simulink model "wt_multi"  (R2022b)
settings: Solver=FixedStepDiscrete  StartTime=0.0  StopTime=10.0  RelTol=1e-3
PreLoadFcn:
  | addpath('/nfs/ug/homes-1/z/zha13325/ece1718/a2_k/a2_hw/hdlimport/wt_multi');
libraries: simulink x2808, hdlsllib x1459
(part 1 of 22)
CloseFcn:
  | addpath('/nfs/ug/homes-1/z/zha13325/ece1718/a2_k/a2_hw/hdlimport/wt_multi');
  | rmpath('/nfs/ug/homes-1/z/zha13325/ece1718/a2_k/a2_hw/hdlimport/wt_multi');
settings Model: DataTypeOverride=Off  Creator=zha13325  LastModifiedBy=zhangjx
settings OptimizationCC: BlockReduction=off  ConditionallyExecuteInputs=off  DefaultParameterBehavior=Inlined
settings DebuggingCC: AlgebraicLoopMsg=error  InheritedTsInSrcMsg=none  SingleTaskRateTransMsg=error  UnconnectedInputMsg=warning  UnconnectedOutputMsg=warning  UnconnectedLineMsg=warning
settings HardwareCC: ProdBitPerPointer=32  ProdBitPerSizeT=32  ProdBitPerPtrDiffT=32  ProdLargestAtomicFloat=None  ProdIntDivRoundTo=Undefined  ProdEndianess=Unspecified  ProdWordSize=32  ProdHWDeviceType=ASIC/FPGA->ASIC/FPGA  TargetBitPerLong=64  TargetBitPerPointer=64  TargetBitPerSizeT=64  TargetBitPerPtrDiffT=64  TargetLongLongMode=on  TargetIntDivRoundTo=Zero  TargetEndianess=LittleEndian  TargetWordSize=64  TargetHWDeviceType=Custom Processor->MATLAB Host Computer  ProdEqTarget=off
settings ModelReferenceCC: EnableRefExpFcnMdlSchedulingChecks=on
settings RTWCC: DLArmComputeVersion=19.05

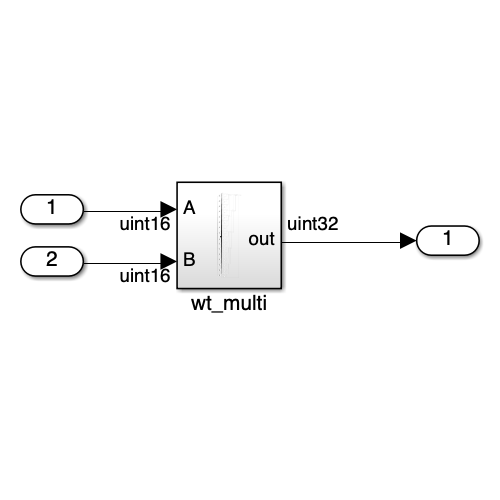
[thumbnail: Simulink's stored preview of the top-level diagram]
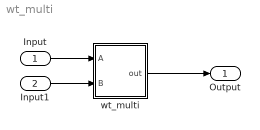
== system wt_multi ==
  Input : Inport
  Input1 : Inport  Port=2
  wt_multi : Subsystem
  Output : Outport
  wires:
  Input/1 -> wt_multi/1(A)
  Input1/1 -> wt_multi/2(B)
  wt_multi/1(out) -> Output/1

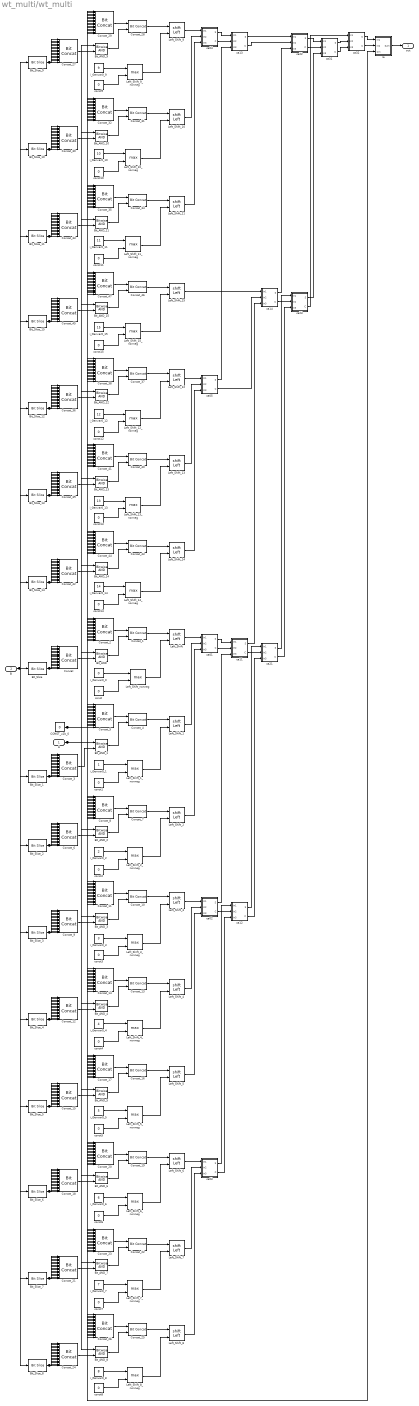
== system wt_multi/wt_multi ==
  A : Inport  OutDataTypeStr=uint16  SampleTime=-1
  B : Inport  Port=2  OutDataTypeStr=uint16  SampleTime=-1
  Bit_AND : simulink/Logic and Bit Operations/Bitwise Operator  logicop=AND  UseBitMask=off  NumInputPorts=2  BitMask=double(0)  BitMaskRealWorld=Real World Value
  Bit_AND_{1..15} (15 alike) : simulink/Logic and Bit Operations/Bitwise Operator  logicop=AND  UseBitMask=off  NumInputPorts=2  BitMask=double(0)  BitMaskRealWorld=Real World Value
  Bit_Slice : hdlsllib/Logic and Bit Operations/Bit Slice  lidx=double(0)  ridx=double(0)
  Bit_Slice_1 : hdlsllib/Logic and Bit Operations/Bit Slice  lidx=double(1)  ridx=double(1)
  Bit_Slice_10 : hdlsllib/Logic and Bit Operations/Bit Slice  lidx=double(10)  ridx=double(10)
  Bit_Slice_11 : hdlsllib/Logic and Bit Operations/Bit Slice  lidx=double(11)  ridx=double(11)
  Bit_Slice_12 : hdlsllib/Logic and Bit Operations/Bit Slice  lidx=double(12)  ridx=double(12)
  Bit_Slice_13 : hdlsllib/Logic and Bit Operations/Bit Slice  lidx=double(13)  ridx=double(13)
  Bit_Slice_14 : hdlsllib/Logic and Bit Operations/Bit Slice  lidx=double(14)  ridx=double(14)
  Bit_Slice_15 : hdlsllib/Logic and Bit Operations/Bit Slice  lidx=double(15)  ridx=double(15)
  Bit_Slice_2 : hdlsllib/Logic and Bit Operations/Bit Slice  lidx=double(2)  ridx=double(2)
  Bit_Slice_3 : hdlsllib/Logic and Bit Operations/Bit Slice  lidx=double(3)  ridx=double(3)
  Bit_Slice_4 : hdlsllib/Logic and Bit Operations/Bit Slice  lidx=double(4)  ridx=double(4)
  Bit_Slice_5 : hdlsllib/Logic and Bit Operations/Bit Slice  lidx=double(5)  ridx=double(5)
  Bit_Slice_6 : hdlsllib/Logic and Bit Operations/Bit Slice  lidx=double(6)  ridx=double(6)
  Bit_Slice_7 : hdlsllib/Logic and Bit Operations/Bit Slice  lidx=double(7)  ridx=double(7)
  Bit_Slice_8 : hdlsllib/Logic and Bit Operations/Bit Slice  lidx=double(8)  ridx=double(8)
  Bit_Slice_9 : hdlsllib/Logic and Bit Operations/Bit Slice  lidx=double(9)  ridx=double(9)
  CONST_u1b_0 : Constant  Value=0  OutDataTypeStr=fixdt(0, 1, 0)  SampleTime=-1
  Concat : hdlsllib/Logic and Bit Operations/Bit Concat  numInputs=16
  Concat_{1,4,7,10,13,16,19,22,25,28,31,34,37,40,43,46} (16 alike) : hdlsllib/Logic and Bit Operations/Bit Concat  numInputs=2
  Concat_{2..3,5..6,8..9,11..12,14..15,17..18,20..21,23..24,26..27,29..30,32..33,35..36,38..39,41..42,44..45,47} (31 alike) : hdlsllib/Logic and Bit Operations/Bit Concat  numInputs=16
  Left_Shift : ArithShift  BitShiftNumberSource=Input port  BitShiftDirection=Left
      settings: InputPortMap=u0,p1
  Left_Shift_{1..15} (15 alike) : ArithShift  BitShiftNumberSource=Input port  BitShiftDirection=Left
      settings: InputPortMap=u0,p1
  Left_Shift_10_nonneg : MinMax  Function=max  Inputs=2
  Left_Shift_11_nonneg : MinMax  Function=max  Inputs=2
  Left_Shift_12_nonneg : MinMax  Function=max  Inputs=2
  Left_Shift_13_nonneg : MinMax  Function=max  Inputs=2
  Left_Shift_14_nonneg : MinMax  Function=max  Inputs=2
  Left_Shift_15_nonneg : MinMax  Function=max  Inputs=2
  Left_Shift_1_nonneg : MinMax  Function=max  Inputs=2
  Left_Shift_2_nonneg : MinMax  Function=max  Inputs=2
  Left_Shift_3_nonneg : MinMax  Function=max  Inputs=2
  Left_Shift_4_nonneg : MinMax  Function=max  Inputs=2
  Left_Shift_5_nonneg : MinMax  Function=max  Inputs=2
  Left_Shift_6_nonneg : MinMax  Function=max  Inputs=2
  Left_Shift_7_nonneg : MinMax  Function=max  Inputs=2
  Left_Shift_8_nonneg : MinMax  Function=max  Inputs=2
  Left_Shift_9_nonneg : MinMax  Function=max  Inputs=2
  Left_Shift_nonneg : MinMax  Function=max  Inputs=2
  ca01 : Subsystem
  ca02 : Subsystem
  ca03 : Subsystem
  ca04 : Subsystem
  ca05 : Subsystem
  ca11 : Subsystem
  ca12 : Subsystem
  ca13 : Subsystem
  ca14 : Subsystem
  ca21 : Subsystem
  ca22 : Subsystem
  ca23 : Subsystem
  ca31 : Subsystem
  ca32 : Subsystem
  const{,1..15} (16 alike) : Constant  Value=0  OutDataTypeStr=int32  SampleTime=-1
  i_Genvar0_0 : Constant  Value=0  OutDataTypeStr=int32  SampleTime=-1
  i_Genvar0_1 : Constant  OutDataTypeStr=int32  SampleTime=-1
  i_Genvar0_10 : Constant  Value=10  OutDataTypeStr=int32  SampleTime=-1
  i_Genvar0_11 : Constant  Value=11  OutDataTypeStr=int32  SampleTime=-1
  i_Genvar0_12 : Constant  Value=12  OutDataTypeStr=int32  SampleTime=-1
  i_Genvar0_13 : Constant  Value=13  OutDataTypeStr=int32  SampleTime=-1
  i_Genvar0_14 : Constant  Value=14  OutDataTypeStr=int32  SampleTime=-1
  i_Genvar0_15 : Constant  Value=15  OutDataTypeStr=int32  SampleTime=-1
  i_Genvar0_2 : Constant  Value=2  OutDataTypeStr=int32  SampleTime=-1
  i_Genvar0_3 : Constant  Value=3  OutDataTypeStr=int32  SampleTime=-1
  i_Genvar0_4 : Constant  Value=4  OutDataTypeStr=int32  SampleTime=-1
  i_Genvar0_5 : Constant  Value=5  OutDataTypeStr=int32  SampleTime=-1
  i_Genvar0_6 : Constant  Value=6  OutDataTypeStr=int32  SampleTime=-1
  i_Genvar0_7 : Constant  Value=7  OutDataTypeStr=int32  SampleTime=-1
  i_Genvar0_8 : Constant  Value=8  OutDataTypeStr=int32  SampleTime=-1
  i_Genvar0_9 : Constant  Value=9  OutDataTypeStr=int32  SampleTime=-1
  ra : Subsystem
  out : Outport  OutDataTypeStr=uint32  SampleTime=-1
  wires:
  B/1 -> Bit_Slice_15/1, Bit_Slice_14/1, Bit_Slice_13/1, Bit_Slice_12/1, Bit_Slice_11/1, Bit_Slice_10/1, Bit_Slice_9/1, Bit_Slice_8/1, Bit_Slice_7/1, Bit_Slice_6/1, Bit_Slice_5/1, Bit_Slice_4/1, Bit_Slice_3/1, Bit_Slice_2/1, Bit_Slice_1/1, Bit_Slice/1
  Bit_Slice/1 -> Concat/16, Concat/15, Concat/14, Concat/13, Concat/12, Concat/11, Concat/10, Concat/9, Concat/8, Concat/7, Concat/6, Concat/5, Concat/4, Concat/3, Concat/2, Concat/1
  CONST_u1b_0/1 -> Concat_47/16, Concat_47/15, Concat_47/14, Concat_47/13, Concat_47/12, Concat_47/11, Concat_47/10, Concat_47/9, Concat_47/8, Concat_47/7, Concat_47/6, Concat_47/5, Concat_47/4, Concat_47/3, Concat_47/2, Concat_47/1, Concat_44/16, Concat_44/15, Concat_44/14, Concat_44/13, Concat_44/12, Concat_44/11, Concat_44/10, Concat_44/9, Concat_44/8, Concat_44/7, Concat_44/6, Concat_44/5, Concat_44/4, Concat_44/3, Concat_44/2, Concat_44/1, Concat_41/16, Concat_41/15, Concat_41/14, Concat_41/13, Concat_41/12, Concat_41/11, Concat_41/10, Concat_41/9, Concat_41/8, Concat_41/7, Concat_41/6, Concat_41/5, Concat_41/4, Concat_41/3, Concat_41/2, Concat_41/1, Concat_38/16, Concat_38/15, Concat_38/14, Concat_38/13, Concat_38/12, Concat_38/11, Concat_38/10, Concat_38/9, Concat_38/8, Concat_38/7, Concat_38/6, Concat_38/5, Concat_38/4, Concat_38/3, Concat_38/2, Concat_38/1, Concat_35/16, Concat_35/15, Concat_35/14, Concat_35/13, Concat_35/12, Concat_35/11, Concat_35/10, Concat_35/9, Concat_35/8, Concat_35/7, Concat_35/6, Concat_35/5, Concat_35/4, Concat_35/3, Concat_35/2, Concat_35/1, Concat_32/16, Concat_32/15, Concat_32/14, Concat_32/13, Concat_32/12, Concat_32/11, Concat_32/10, Concat_32/9, Concat_32/8, Concat_32/7, Concat_32/6, Concat_32/5, Concat_32/4, Concat_32/3, Concat_32/2, Concat_32/1, Concat_29/16, Concat_29/15, Concat_29/14, Concat_29/13, Concat_29/12, Concat_29/11, Concat_29/10, Concat_29/9, Concat_29/8, Concat_29/7, Concat_29/6, Concat_29/5, Concat_29/4, Concat_29/3, Concat_29/2, Concat_29/1, Concat_26/16, Concat_26/15, Concat_26/14, Concat_26/13, Concat_26/12, Concat_26/11, Concat_26/10, Concat_26/9, Concat_26/8, Concat_26/7, Concat_26/6, Concat_26/5, Concat_26/4, Concat_26/3, Concat_26/2, Concat_26/1, Concat_23/16, Concat_23/15, Concat_23/14, Concat_23/13, Concat_23/12, Concat_23/11, Concat_23/10, Concat_23/9, Concat_23/8, Concat_23/7, Concat_23/6, Concat_23/5, Concat_23/4, Concat_23/3, Concat_23/2, Concat_23/1, Concat_20/16, Concat_20/15, Concat_20/14, Concat_20/13, Concat_20/12, Concat_20/11, Concat_20/10, Concat_20/9, Concat_20/8, Concat_20/7, Concat_20/6, Concat_20/5, Concat_20/4, Concat_20/3, Concat_20/2, Concat_20/1, Concat_17/16, Concat_17/15, Concat_17/14, Concat_17/13, Concat_17/12, Concat_17/11, Concat_17/10, Concat_17/9, Concat_17/8, Concat_17/7, Concat_17/6, Concat_17/5, Concat_17/4, Concat_17/3, Concat_17/2, Concat_17/1, Concat_14/16, Concat_14/15, Concat_14/14, Concat_14/13, Concat_14/12, Concat_14/11, Concat_14/10, Concat_14/9, Concat_14/8, Concat_14/7, Concat_14/6, Concat_14/5, Concat_14/4, Concat_14/3, Concat_14/2, Concat_14/1, Concat_11/16, Concat_11/15, Concat_11/14, Concat_11/13, Concat_11/12, Concat_11/11, Concat_11/10, Concat_11/9, Concat_11/8, Concat_11/7, Concat_11/6, Concat_11/5, Concat_11/4, Concat_11/3, Concat_11/2, Concat_11/1, Concat_8/16, Concat_8/15, Concat_8/14, Concat_8/13, Concat_8/12, Concat_8/11, Concat_8/10, Concat_8/9, Concat_8/8, Concat_8/7, Concat_8/6, Concat_8/5, Concat_8/4, Concat_8/3, Concat_8/2, Concat_8/1, Concat_5/16, Concat_5/15, Concat_5/14, Concat_5/13, Concat_5/12, Concat_5/11, Concat_5/10, Concat_5/9, Concat_5/8, Concat_5/7, Concat_5/6, Concat_5/5, Concat_5/4, Concat_5/3, Concat_5/2, Concat_5/1, Concat_2/16, Concat_2/15, Concat_2/14, Concat_2/13, Concat_2/12, Concat_2/11, Concat_2/10, Concat_2/9, Concat_2/8, Concat_2/7, Concat_2/6, Concat_2/5, Concat_2/4, Concat_2/3, Concat_2/2, Concat_2/1, ra/3(Cin)
  Bit_Slice_1/1 -> Concat_3/16, Concat_3/15, Concat_3/14, Concat_3/13, Concat_3/12, Concat_3/11, Concat_3/10, Concat_3/9, Concat_3/8, Concat_3/7, Concat_3/6, Concat_3/5, Concat_3/4, Concat_3/3, Concat_3/2, Concat_3/1
  Bit_Slice_3/1 -> Concat_9/16, Concat_9/15, Concat_9/14, Concat_9/13, Concat_9/12, Concat_9/11, Concat_9/10, Concat_9/9, Concat_9/8, Concat_9/7, Concat_9/6, Concat_9/5, Concat_9/4, Concat_9/3, Concat_9/2, Concat_9/1
  Bit_Slice_5/1 -> Concat_15/16, Concat_15/15, Concat_15/14, Concat_15/13, Concat_15/12, Concat_15/11, Concat_15/10, Concat_15/9, Concat_15/8, Concat_15/7, Concat_15/6, Concat_15/5, Concat_15/4, Concat_15/3, Concat_15/2, Concat_15/1
  Bit_Slice_6/1 -> Concat_18/16, Concat_18/15, Concat_18/14, Concat_18/13, Concat_18/12, Concat_18/11, Concat_18/10, Concat_18/9, Concat_18/8, Concat_18/7, Concat_18/6, Concat_18/5, Concat_18/4, Concat_18/3, Concat_18/2, Concat_18/1
  Concat_39/1 -> Bit_AND_13/2
  Left_Shift_15/1 -> ca14/1(in1)
  const10/1 -> Left_Shift_10_nonneg/2
  Left_Shift_1_nonneg/1 -> Left_Shift_1/2
  Left_Shift_5_nonneg/1 -> Left_Shift_5/2
  i_Genvar0_13/1 -> Left_Shift_13_nonneg/1
  Concat_10/1 -> Left_Shift_3/1
  Bit_AND_14/1 -> Concat_43/2
  i_Genvar0_8/1 -> Left_Shift_8_nonneg/1
  Concat_43/1 -> Left_Shift_14/1
  i_Genvar0_15/1 -> Left_Shift_15_nonneg/1
  Concat_32/1 -> Concat_31/1
  Concat_45/1 -> Bit_AND_15/2
  Concat_12/1 -> Bit_AND_4/2
  Bit_AND_15/1 -> Concat_46/2
  Concat_47/1 -> Concat_46/1
  ca02/2(C) -> ca12/2(in2)
  ca04/1(S) -> ca13/1(in1)
  ca03/2(C) -> ca12/3(in3)
  ca05/1(S) -> ca13/3(in3)
  A/1 -> Bit_AND_15/1, Bit_AND_14/1, Bit_AND_13/1, Bit_AND_12/1, Bit_AND_11/1, Bit_AND_10/1, Bit_AND_9/1, Bit_AND_8/1, Bit_AND_7/1, Bit_AND_6/1, Bit_AND_5/1, Bit_AND_4/1, Bit_AND_3/1, Bit_AND_2/1, Bit_AND_1/1, Bit_AND/1
  Concat_13/1 -> Left_Shift_4/1
  ca11/2(C) -> ca21/2(in2)
  ca22/1(S) -> ca31/1(in1)
  ca12/2(C) -> ca21/3(in3)
  ca01/2(C) -> ca11/2(in2)
  ca23/1(S) -> ca31/3(in3)
  ca32/1(S) -> ra/1(in1)
  ca13/1(S) -> ca22/1(in1)
  ca13/2(C) -> ca22/2(in2)
  ca32/2(C) -> ra/2(in2)
  ca14/2(C) -> ca23/2(in2)
  Left_Shift_11_nonneg/1 -> Left_Shift_11/2
  Concat_41/1 -> Concat_40/1
  Concat_25/1 -> Left_Shift_8/1
  ca03/1(S) -> ca12/1(in1)
  ca05/2(C) -> ca14/2(in2)
  ca22/2(C) -> ca31/2(in2)
  Concat_15/1 -> Bit_AND_5/2
  Left_Shift_14/1 -> ca05/3(in3)
  ca01/1(S) -> ca11/1(in1)
  i_Genvar0_6/1 -> Left_Shift_6_nonneg/1
  Concat_3/1 -> Bit_AND_1/2
  ca02/1(S) -> ca11/3(in3)
  Concat_24/1 -> Bit_AND_8/2
  const5/1 -> Left_Shift_5_nonneg/2
  ca11/1(S) -> ca14/3(in3)
  ca23/2(C) -> ca32/1(in1)
  Concat_27/1 -> Bit_AND_9/2
  i_Genvar0_2/1 -> Left_Shift_2_nonneg/1
  ca14/1(S) -> ca22/3(in3)
  const13/1 -> Left_Shift_13_nonneg/2
  Left_Shift_8/1 -> ca03/3(in3)
  const9/1 -> Left_Shift_9_nonneg/2
  const8/1 -> Left_Shift_8_nonneg/2
  ca31/1(S) -> ca32/2(in2)
  Concat_14/1 -> Concat_13/1
  Concat_21/1 -> Bit_AND_7/2
  ca12/1(S) -> ca21/1(in1)
  const11/1 -> Left_Shift_11_nonneg/2
  i_Genvar0_3/1 -> Left_Shift_3_nonneg/1
  Bit_Slice_2/1 -> Concat_6/16, Concat_6/15, Concat_6/14, Concat_6/13, Concat_6/12, Concat_6/11, Concat_6/10, Concat_6/9, Concat_6/8, Concat_6/7, Concat_6/6, Concat_6/5, Concat_6/4, Concat_6/3, Concat_6/2, Concat_6/1
  const2/1 -> Left_Shift_2_nonneg/2
  const6/1 -> Left_Shift_6_nonneg/2
  Concat_11/1 -> Concat_10/1
  i_Genvar0_5/1 -> Left_Shift_5_nonneg/1
  const12/1 -> Left_Shift_12_nonneg/2
  Left_Shift_8_nonneg/1 -> Left_Shift_8/2
  Left_Shift_15_nonneg/1 -> Left_Shift_15/2
  const3/1 -> Left_Shift_3_nonneg/2
  Left_Shift_13/1 -> ca05/2(in2)
  Left_Shift_3_nonneg/1 -> Left_Shift_3/2
  const15/1 -> Left_Shift_15_nonneg/2
  Concat_44/1 -> Concat_43/1
  Concat_7/1 -> Left_Shift_2/1
  ca21/1(S) -> ca23/1(in1)
  Left_Shift_9_nonneg/1 -> Left_Shift_9/2
  Left_Shift_7_nonneg/1 -> Left_Shift_7/2
  ca04/2(C) -> ca13/2(in2)
  Left_Shift_12_nonneg/1 -> Left_Shift_12/2
  Bit_Slice_11/1 -> Concat_33/16, Concat_33/15, Concat_33/14, Concat_33/13, Concat_33/12, Concat_33/11, Concat_33/10, Concat_33/9, Concat_33/8, Concat_33/7, Concat_33/6, Concat_33/5, Concat_33/4, Concat_33/3, Concat_33/2, Concat_33/1
  Left_Shift_6_nonneg/1 -> Left_Shift_6/2
  Bit_AND_11/1 -> Concat_34/2
  Bit_AND_13/1 -> Concat_40/2
  i_Genvar0_14/1 -> Left_Shift_14_nonneg/1
  const4/1 -> Left_Shift_4_nonneg/2
  Bit_Slice_15/1 -> Concat_45/16, Concat_45/15, Concat_45/14, Concat_45/13, Concat_45/12, Concat_45/11, Concat_45/10, Concat_45/9, Concat_45/8, Concat_45/7, Concat_45/6, Concat_45/5, Concat_45/4, Concat_45/3, Concat_45/2, Concat_45/1
  const14/1 -> Left_Shift_14_nonneg/2
  const7/1 -> Left_Shift_7_nonneg/2
  const1/1 -> Left_Shift_1_nonneg/2
  Concat_46/1 -> Left_Shift_15/1
  Left_Shift_2_nonneg/1 -> Left_Shift_2/2
  i_Genvar0_11/1 -> Left_Shift_11_nonneg/1
  Left_Shift_13_nonneg/1 -> Left_Shift_13/2
  Concat_33/1 -> Bit_AND_11/2
  const/1 -> Left_Shift_nonneg/2
  ca31/2(C) -> ca32/3(in3)
  Concat_28/1 -> Left_Shift_9/1
  Left_Shift_nonneg/1 -> Left_Shift/2
  i_Genvar0_7/1 -> Left_Shift_7_nonneg/1
  Concat_37/1 -> Left_Shift_12/1
  Concat_9/1 -> Bit_AND_3/2
  Bit_AND_12/1 -> Concat_37/2
  Left_Shift/1 -> ca01/1(in1)
  Concat_36/1 -> Bit_AND_12/2
  Left_Shift_12/1 -> ca05/1(in1)
  i_Genvar0_12/1 -> Left_Shift_12_nonneg/1
  Bit_AND_5/1 -> Concat_16/2
  Left_Shift_11/1 -> ca04/3(in3)
  Concat_34/1 -> Left_Shift_11/1
  Concat_35/1 -> Concat_34/1
  Concat_29/1 -> Concat_28/1
  Left_Shift_10/1 -> ca04/2(in2)
  Bit_AND_7/1 -> Concat_22/2
  Concat_18/1 -> Bit_AND_6/2
  Concat_31/1 -> Left_Shift_10/1
  Bit_Slice_10/1 -> Concat_30/16, Concat_30/15, Concat_30/14, Concat_30/13, Concat_30/12, Concat_30/11, Concat_30/10, Concat_30/9, Concat_30/8, Concat_30/7, Concat_30/6, Concat_30/5, Concat_30/4, Concat_30/3, Concat_30/2, Concat_30/1
  Left_Shift_3/1 -> ca02/1(in1)
  Concat_30/1 -> Bit_AND_10/2
  i_Genvar0_10/1 -> Left_Shift_10_nonneg/1
  Left_Shift_9/1 -> ca04/1(in1)
  Bit_AND_9/1 -> Concat_28/2
  Left_Shift_10_nonneg/1 -> Left_Shift_10/2
  Bit_AND_4/1 -> Concat_13/2
  i_Genvar0_4/1 -> Left_Shift_4_nonneg/1
  i_Genvar0_9/1 -> Left_Shift_9_nonneg/1
  Concat_26/1 -> Concat_25/1
  Bit_AND_8/1 -> Concat_25/2
  Bit_Slice_4/1 -> Concat_12/16, Concat_12/15, Concat_12/14, Concat_12/13, Concat_12/12, Concat_12/11, Concat_12/10, Concat_12/9, Concat_12/8, Concat_12/7, Concat_12/6, Concat_12/5, Concat_12/4, Concat_12/3, Concat_12/2, Concat_12/1
  Left_Shift_7/1 -> ca03/2(in2)
  Concat_22/1 -> Left_Shift_7/1
  Concat_23/1 -> Concat_22/1
  Left_Shift_6/1 -> ca03/1(in1)
  Concat_19/1 -> Left_Shift_6/1
  ca21/2(C) -> ca23/3(in3)
  Concat_20/1 -> Concat_19/1
  Bit_AND_6/1 -> Concat_19/2
  Left_Shift_5/1 -> ca02/3(in3)
  Concat_8/1 -> Concat_7/1
  Concat_16/1 -> Left_Shift_5/1
  Left_Shift_4/1 -> ca02/2(in2)
  Bit_AND_10/1 -> Concat_31/2
  Bit_AND_3/1 -> Concat_10/2
  Left_Shift_2/1 -> ca01/3(in3)
  Concat_42/1 -> Bit_AND_14/2
  Bit_AND_2/1 -> Concat_7/2
  Concat_6/1 -> Bit_AND_2/2
  Concat_5/1 -> Concat_4/1
  Left_Shift_1/1 -> ca01/2(in2)
  Left_Shift_14_nonneg/1 -> Left_Shift_14/2
  Bit_AND_1/1 -> Concat_4/2
  i_Genvar0_1/1 -> Left_Shift_1_nonneg/1
  Concat_40/1 -> Left_Shift_13/1
  Concat_1/1 -> Left_Shift/1
  Concat_17/1 -> Concat_16/1
  Concat_2/1 -> Concat_1/1
  Bit_AND/1 -> Concat_1/2
  Concat/1 -> Bit_AND/2
  Concat_4/1 -> Left_Shift_1/1
  i_Genvar0_0/1 -> Left_Shift_nonneg/1
  ra/1(Sum) -> out/1
  Left_Shift_4_nonneg/1 -> Left_Shift_4/2
  Concat_38/1 -> Concat_37/1
  Bit_Slice_13/1 -> Concat_39/16, Concat_39/15, Concat_39/14, Concat_39/13, Concat_39/12, Concat_39/11, Concat_39/10, Concat_39/9, Concat_39/8, Concat_39/7, Concat_39/6, Concat_39/5, Concat_39/4, Concat_39/3, Concat_39/2, Concat_39/1
  Bit_Slice_14/1 -> Concat_42/16, Concat_42/15, Concat_42/14, Concat_42/13, Concat_42/12, Concat_42/11, Concat_42/10, Concat_42/9, Concat_42/8, Concat_42/7, Concat_42/6, Concat_42/5, Concat_42/4, Concat_42/3, Concat_42/2, Concat_42/1
  Bit_Slice_12/1 -> Concat_36/16, Concat_36/15, Concat_36/14, Concat_36/13, Concat_36/12, Concat_36/11, Concat_36/10, Concat_36/9, Concat_36/8, Concat_36/7, Concat_36/6, Concat_36/5, Concat_36/4, Concat_36/3, Concat_36/2, Concat_36/1
  Bit_Slice_9/1 -> Concat_27/16, Concat_27/15, Concat_27/14, Concat_27/13, Concat_27/12, Concat_27/11, Concat_27/10, Concat_27/9, Concat_27/8, Concat_27/7, Concat_27/6, Concat_27/5, Concat_27/4, Concat_27/3, Concat_27/2, Concat_27/1
  Bit_Slice_8/1 -> Concat_24/16, Concat_24/15, Concat_24/14, Concat_24/13, Concat_24/12, Concat_24/11, Concat_24/10, Concat_24/9, Concat_24/8, Concat_24/7, Concat_24/6, Concat_24/5, Concat_24/4, Concat_24/3, Concat_24/2, Concat_24/1
  Bit_Slice_7/1 -> Concat_21/16, Concat_21/15, Concat_21/14, Concat_21/13, Concat_21/12, Concat_21/11, Concat_21/10, Concat_21/9, Concat_21/8, Concat_21/7, Concat_21/6, Concat_21/5, Concat_21/4, Concat_21/3, Concat_21/2, Concat_21/1

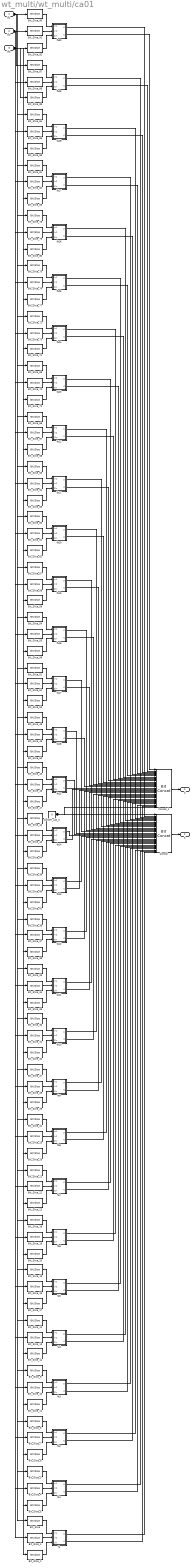
== system wt_multi/wt_multi/ca01 ==
  in1 : Inport  OutDataTypeStr=uint32  SampleTime=-1
  in2 : Inport  Port=2  OutDataTypeStr=uint32  SampleTime=-1
  in3 : Inport  Port=3  OutDataTypeStr=uint32  SampleTime=-1
  Bit_Slice : hdlsllib/Logic and Bit Operations/Bit Slice  lidx=double(0)  ridx=double(0)
  Bit_Slice_1 : hdlsllib/Logic and Bit Operations/Bit Slice  lidx=double(0)  ridx=double(0)
  Bit_Slice_10 : hdlsllib/Logic and Bit Operations/Bit Slice  lidx=double(3)  ridx=double(3)
  Bit_Slice_11 : hdlsllib/Logic and Bit Operations/Bit Slice  lidx=double(3)  ridx=double(3)
  Bit_Slice_12 : hdlsllib/Logic and Bit Operations/Bit Slice  lidx=double(4)  ridx=double(4)
  Bit_Slice_13 : hdlsllib/Logic and Bit Operations/Bit Slice  lidx=double(4)  ridx=double(4)
  Bit_Slice_14 : hdlsllib/Logic and Bit Operations/Bit Slice  lidx=double(4)  ridx=double(4)
  Bit_Slice_15 : hdlsllib/Logic and Bit Operations/Bit Slice  lidx=double(5)  ridx=double(5)
  Bit_Slice_16 : hdlsllib/Logic and Bit Operations/Bit Slice  lidx=double(5)  ridx=double(5)
  Bit_Slice_17 : hdlsllib/Logic and Bit Operations/Bit Slice  lidx=double(5)  ridx=double(5)
  Bit_Slice_18 : hdlsllib/Logic and Bit Operations/Bit Slice  lidx=double(6)  ridx=double(6)
  Bit_Slice_19 : hdlsllib/Logic and Bit Operations/Bit Slice  lidx=double(6)  ridx=double(6)
  Bit_Slice_2 : hdlsllib/Logic and Bit Operations/Bit Slice  lidx=double(0)  ridx=double(0)
  Bit_Slice_20 : hdlsllib/Logic and Bit Operations/Bit Slice  lidx=double(6)  ridx=double(6)
  Bit_Slice_21 : hdlsllib/Logic and Bit Operations/Bit Slice  lidx=double(7)  ridx=double(7)
  Bit_Slice_22 : hdlsllib/Logic and Bit Operations/Bit Slice  lidx=double(7)  ridx=double(7)
  Bit_Slice_23 : hdlsllib/Logic and Bit Operations/Bit Slice  lidx=double(7)  ridx=double(7)
  Bit_Slice_24 : hdlsllib/Logic and Bit Operations/Bit Slice  lidx=double(8)  ridx=double(8)
  Bit_Slice_25 : hdlsllib/Logic and Bit Operations/Bit Slice  lidx=double(8)  ridx=double(8)
  Bit_Slice_26 : hdlsllib/Logic and Bit Operations/Bit Slice  lidx=double(8)  ridx=double(8)
  Bit_Slice_27 : hdlsllib/Logic and Bit Operations/Bit Slice  lidx=double(9)  ridx=double(9)
  Bit_Slice_28 : hdlsllib/Logic and Bit Operations/Bit Slice  lidx=double(9)  ridx=double(9)
  Bit_Slice_29 : hdlsllib/Logic and Bit Operations/Bit Slice  lidx=double(9)  ridx=double(9)
  Bit_Slice_3 : hdlsllib/Logic and Bit Operations/Bit Slice  lidx=double(1)  ridx=double(1)
  Bit_Slice_30 : hdlsllib/Logic and Bit Operations/Bit Slice  lidx=double(10)  ridx=double(10)
  Bit_Slice_31 : hdlsllib/Logic and Bit Operations/Bit Slice  lidx=double(10)  ridx=double(10)
  Bit_Slice_32 : hdlsllib/Logic and Bit Operations/Bit Slice  lidx=double(10)  ridx=double(10)
  Bit_Slice_33 : hdlsllib/Logic and Bit Operations/Bit Slice  lidx=double(11)  ridx=double(11)
  Bit_Slice_34 : hdlsllib/Logic and Bit Operations/Bit Slice  lidx=double(11)  ridx=double(11)
  Bit_Slice_35 : hdlsllib/Logic and Bit Operations/Bit Slice  lidx=double(11)  ridx=double(11)
  Bit_Slice_36 : hdlsllib/Logic and Bit Operations/Bit Slice  lidx=double(12)  ridx=double(12)
  Bit_Slice_37 : hdlsllib/Logic and Bit Operations/Bit Slice  lidx=double(12)  ridx=double(12)
  Bit_Slice_38 : hdlsllib/Logic and Bit Operations/Bit Slice  lidx=double(12)  ridx=double(12)
  Bit_Slice_39 : hdlsllib/Logic and Bit Operations/Bit Slice  lidx=double(13)  ridx=double(13)
  Bit_Slice_4 : hdlsllib/Logic and Bit Operations/Bit Slice  lidx=double(1)  ridx=double(1)
  Bit_Slice_40 : hdlsllib/Logic and Bit Operations/Bit Slice  lidx=double(13)  ridx=double(13)
  Bit_Slice_41 : hdlsllib/Logic and Bit Operations/Bit Slice  lidx=double(13)  ridx=double(13)
  Bit_Slice_42 : hdlsllib/Logic and Bit Operations/Bit Slice  lidx=double(14)  ridx=double(14)
  Bit_Slice_43 : hdlsllib/Logic and Bit Operations/Bit Slice  lidx=double(14)  ridx=double(14)
  Bit_Slice_44 : hdlsllib/Logic and Bit Operations/Bit Slice  lidx=double(14)  ridx=double(14)
  Bit_Slice_45 : hdlsllib/Logic and Bit Operations/Bit Slice  lidx=double(15)  ridx=double(15)
  Bit_Slice_46 : hdlsllib/Logic and Bit Operations/Bit Slice  lidx=double(15)  ridx=double(15)
  Bit_Slice_47 : hdlsllib/Logic and Bit Operations/Bit Slice  lidx=double(15)  ridx=double(15)
  Bit_Slice_48 : hdlsllib/Logic and Bit Operations/Bit Slice  lidx=double(16)  ridx=double(16)
  Bit_Slice_49 : hdlsllib/Logic and Bit Operations/Bit Slice  lidx=double(16)  ridx=double(16)
  Bit_Slice_5 : hdlsllib/Logic and Bit Operations/Bit Slice  lidx=double(1)  ridx=double(1)
  Bit_Slice_50 : hdlsllib/Logic and Bit Operations/Bit Slice  lidx=double(16)  ridx=double(16)
  Bit_Slice_51 : hdlsllib/Logic and Bit Operations/Bit Slice  lidx=double(17)  ridx=double(17)
  Bit_Slice_52 : hdlsllib/Logic and Bit Operations/Bit Slice  lidx=double(17)  ridx=double(17)
  Bit_Slice_53 : hdlsllib/Logic and Bit Operations/Bit Slice  lidx=double(17)  ridx=double(17)
  Bit_Slice_54 : hdlsllib/Logic and Bit Operations/Bit Slice  lidx=double(18)  ridx=double(18)
  Bit_Slice_55 : hdlsllib/Logic and Bit Operations/Bit Slice  lidx=double(18)  ridx=double(18)
  Bit_Slice_56 : hdlsllib/Logic and Bit Operations/Bit Slice  lidx=double(18)  ridx=double(18)
  Bit_Slice_57 : hdlsllib/Logic and Bit Operations/Bit Slice  lidx=double(19)  ridx=double(19)
  Bit_Slice_58 : hdlsllib/Logic and Bit Operations/Bit Slice  lidx=double(19)  ridx=double(19)
  Bit_Slice_59 : hdlsllib/Logic and Bit Operations/Bit Slice  lidx=double(19)  ridx=double(19)
  Bit_Slice_6 : hdlsllib/Logic and Bit Operations/Bit Slice  lidx=double(2)  ridx=double(2)
  Bit_Slice_60 : hdlsllib/Logic and Bit Operations/Bit Slice  lidx=double(20)  ridx=double(20)
  Bit_Slice_61 : hdlsllib/Logic and Bit Operations/Bit Slice  lidx=double(20)  ridx=double(20)
  Bit_Slice_62 : hdlsllib/Logic and Bit Operations/Bit Slice  lidx=double(20)  ridx=double(20)
  Bit_Slice_63 : hdlsllib/Logic and Bit Operations/Bit Slice  lidx=double(21)  ridx=double(21)
  Bit_Slice_64 : hdlsllib/Logic and Bit Operations/Bit Slice  lidx=double(21)  ridx=double(21)
  Bit_Slice_65 : hdlsllib/Logic and Bit Operations/Bit Slice  lidx=double(21)  ridx=double(21)
  Bit_Slice_66 : hdlsllib/Logic and Bit Operations/Bit Slice  lidx=double(22)  ridx=double(22)
  Bit_Slice_67 : hdlsllib/Logic and Bit Operations/Bit Slice  lidx=double(22)  ridx=double(22)
  Bit_Slice_68 : hdlsllib/Logic and Bit Operations/Bit Slice  lidx=double(22)  ridx=double(22)
  Bit_Slice_69 : hdlsllib/Logic and Bit Operations/Bit Slice  lidx=double(23)  ridx=double(23)
  Bit_Slice_7 : hdlsllib/Logic and Bit Operations/Bit Slice  lidx=double(2)  ridx=double(2)
  Bit_Slice_70 : hdlsllib/Logic and Bit Operations/Bit Slice  lidx=double(23)  ridx=double(23)
  Bit_Slice_71 : hdlsllib/Logic and Bit Operations/Bit Slice  lidx=double(23)  ridx=double(23)
  Bit_Slice_72 : hdlsllib/Logic and Bit Operations/Bit Slice  lidx=double(24)  ridx=double(24)
  Bit_Slice_73 : hdlsllib/Logic and Bit Operations/Bit Slice  lidx=double(24)  ridx=double(24)
  Bit_Slice_74 : hdlsllib/Logic and Bit Operations/Bit Slice  lidx=double(24)  ridx=double(24)
  Bit_Slice_75 : hdlsllib/Logic and Bit Operations/Bit Slice  lidx=double(25)  ridx=double(25)
  Bit_Slice_76 : hdlsllib/Logic and Bit Operations/Bit Slice  lidx=double(25)  ridx=double(25)
  Bit_Slice_77 : hdlsllib/Logic and Bit Operations/Bit Slice  lidx=double(25)  ridx=double(25)
  Bit_Slice_78 : hdlsllib/Logic and Bit Operations/Bit Slice  lidx=double(26)  ridx=double(26)
  Bit_Slice_79 : hdlsllib/Logic and Bit Operations/Bit Slice  lidx=double(26)  ridx=double(26)
  Bit_Slice_8 : hdlsllib/Logic and Bit Operations/Bit Slice  lidx=double(2)  ridx=double(2)
  Bit_Slice_80 : hdlsllib/Logic and Bit Operations/Bit Slice  lidx=double(26)  ridx=double(26)
  Bit_Slice_81 : hdlsllib/Logic and Bit Operations/Bit Slice  lidx=double(27)  ridx=double(27)
  Bit_Slice_82 : hdlsllib/Logic and Bit Operations/Bit Slice  lidx=double(27)  ridx=double(27)
  Bit_Slice_83 : hdlsllib/Logic and Bit Operations/Bit Slice  lidx=double(27)  ridx=double(27)
  Bit_Slice_84 : hdlsllib/Logic and Bit Operations/Bit Slice  lidx=double(28)  ridx=double(28)
  Bit_Slice_85 : hdlsllib/Logic and Bit Operations/Bit Slice  lidx=double(28)  ridx=double(28)
  Bit_Slice_86 : hdlsllib/Logic and Bit Operations/Bit Slice  lidx=double(28)  ridx=double(28)
  Bit_Slice_87 : hdlsllib/Logic and Bit Operations/Bit Slice  lidx=double(29)  ridx=double(29)
  Bit_Slice_88 : hdlsllib/Logic and Bit Operations/Bit Slice  lidx=double(29)  ridx=double(29)
  Bit_Slice_89 : hdlsllib/Logic and Bit Operations/Bit Slice  lidx=double(29)  ridx=double(29)
  Bit_Slice_9 : hdlsllib/Logic and Bit Operations/Bit Slice  lidx=double(3)  ridx=double(3)
  Bit_Slice_90 : hdlsllib/Logic and Bit Operations/Bit Slice  lidx=double(30)  ridx=double(30)
  Bit_Slice_91 : hdlsllib/Logic and Bit Operations/Bit Slice  lidx=double(30)  ridx=double(30)
  Bit_Slice_92 : hdlsllib/Logic and Bit Operations/Bit Slice  lidx=double(30)  ridx=double(30)
  CONST_u1b_0 : Constant  Value=0  OutDataTypeStr=fixdt(0, 1, 0)  SampleTime=-1
  Concat : hdlsllib/Logic and Bit Operations/Bit Concat  numInputs=32
  Concat_1 : hdlsllib/Logic and Bit Operations/Bit Concat  numInputs=32
  fa : Subsystem
  fa1 : Subsystem
  fa10 : Subsystem
  fa11 : Subsystem
  fa12 : Subsystem
  fa13 : Subsystem
  fa14 : Subsystem
  fa15 : Subsystem
  fa16 : Subsystem
  fa17 : Subsystem
  fa18 : Subsystem
  fa19 : Subsystem
  fa2 : Subsystem
  fa20 : Subsystem
  fa21 : Subsystem
  fa22 : Subsystem
  fa23 : Subsystem
  fa24 : Subsystem
  fa25 : Subsystem
  fa26 : Subsystem
  fa27 : Subsystem
  fa28 : Subsystem
  fa29 : Subsystem
  fa3 : Subsystem
  fa30 : Subsystem
  fa4 : Subsystem
  fa5 : Subsystem
  fa6 : Subsystem
  fa7 : Subsystem
  fa8 : Subsystem
  fa9 : Subsystem
  S : Outport  OutDataTypeStr=uint32  SampleTime=-1
  C : Outport  Port=2  OutDataTypeStr=uint32  SampleTime=-1
  wires:
  in1/1 -> Bit_Slice_90/1, Bit_Slice_87/1, Bit_Slice_84/1, Bit_Slice_81/1, Bit_Slice_78/1, Bit_Slice_75/1, Bit_Slice_72/1, Bit_Slice_69/1, Bit_Slice_66/1, Bit_Slice_63/1, Bit_Slice_60/1, Bit_Slice_57/1, Bit_Slice_54/1, Bit_Slice_51/1, Bit_Slice_48/1, Bit_Slice_45/1, Bit_Slice_42/1, Bit_Slice_39/1, Bit_Slice_36/1, Bit_Slice_33/1, Bit_Slice_30/1, Bit_Slice_27/1, Bit_Slice_24/1, Bit_Slice_21/1, Bit_Slice_18/1, Bit_Slice_15/1, Bit_Slice_12/1, Bit_Slice_9/1, Bit_Slice_6/1, Bit_Slice_3/1, Bit_Slice/1
  Concat/1 -> S/1
  Bit_Slice_1/1 -> fa/2(in2)
  fa/1(S) -> Concat/32
  Bit_Slice_5/1 -> fa1/3(Cin)
  fa1/1(S) -> Concat/31
  fa1/2(C) -> Concat_1/30
  Bit_Slice_7/1 -> fa2/2(in2)
  Bit_Slice_8/1 -> fa2/3(Cin)
  Bit_Slice_10/1 -> fa3/2(in2)
  fa3/2(C) -> Concat_1/28
  Bit_Slice_9/1 -> fa3/1(in1)
  Bit_Slice_12/1 -> fa4/1(in1)
  Bit_Slice_13/1 -> fa4/2(in2)
  Bit_Slice_14/1 -> fa4/3(Cin)
  fa4/2(C) -> Concat_1/27
  Bit_Slice_15/1 -> fa5/1(in1)
  Bit_Slice_16/1 -> fa5/2(in2)
  Bit_Slice_17/1 -> fa5/3(Cin)
  fa5/1(S) -> Concat/27
  Bit_Slice_19/1 -> fa6/2(in2)
  fa5/2(C) -> Concat_1/26
  fa6/2(C) -> Concat_1/25
  Bit_Slice_21/1 -> fa7/1(in1)
  Bit_Slice_22/1 -> fa7/2(in2)
  Bit_Slice_23/1 -> fa7/3(Cin)
  fa7/1(S) -> Concat/25
  fa/2(C) -> Concat_1/31
  fa3/1(S) -> Concat/29
  Bit_Slice_24/1 -> fa8/1(in1)
  fa8/2(C) -> Concat_1/23
  Bit_Slice_29/1 -> fa9/3(Cin)
  fa6/1(S) -> Concat/26
  fa9/1(S) -> Concat/23
  Bit_Slice_32/1 -> fa10/3(Cin)
  fa10/1(S) -> Concat/22
  Bit_Slice_33/1 -> fa11/1(in1)
  Bit_Slice_35/1 -> fa11/3(Cin)
  fa2/1(S) -> Concat/30
  fa11/2(C) -> Concat_1/20
  Bit_Slice_37/1 -> fa12/2(in2)
  Bit_Slice_25/1 -> fa8/2(in2)
  fa12/1(S) -> Concat/20
  Bit_Slice_40/1 -> fa13/2(in2)
  Bit_Slice_41/1 -> fa13/3(Cin)
  fa2/2(C) -> Concat_1/29
  Bit_Slice_42/1 -> fa14/1(in1)
  Bit_Slice_39/1 -> fa13/1(in1)
  Bit_Slice_44/1 -> fa14/3(Cin)
  fa14/1(S) -> Concat/18
  fa14/2(C) -> Concat_1/17
  Bit_Slice_45/1 -> fa15/1(in1)
  Bit_Slice_2/1 -> fa/3(Cin)
  Bit_Slice_46/1 -> fa15/2(in2)
  Bit_Slice_78/1 -> fa26/1(in1)
  fa30/2(C) -> Concat_1/1
  Bit_Slice_57/1 -> fa19/1(in1)
  Bit_Slice_81/1 -> fa27/1(in1)
  Bit_Slice_77/1 -> fa25/3(Cin)
  Bit_Slice_30/1 -> fa10/1(in1)
  fa26/1(S) -> Concat/6
  fa4/1(S) -> Concat/28
  fa23/2(C) -> Concat_1/8
  Bit_Slice_18/1 -> fa6/1(in1)
  fa12/2(C) -> Concat_1/19
  fa27/1(S) -> Concat/5
  Bit_Slice_34/1 -> fa11/2(in2)
  Bit_Slice_64/1 -> fa21/2(in2)
  Bit_Slice_74/1 -> fa24/3(Cin)
  fa26/2(C) -> Concat_1/5
  Bit_Slice_83/1 -> fa27/3(Cin)
  Bit_Slice_73/1 -> fa24/2(in2)
  Bit_Slice_86/1 -> fa28/3(Cin)
  Bit_Slice_92/1 -> fa30/3(Cin)
  fa29/1(S) -> Concat/3
  CONST_u1b_0/1 -> Concat_1/32, Concat/1
  Bit_Slice_85/1 -> fa28/2(in2)
  fa27/2(C) -> Concat_1/4
  Bit_Slice_3/1 -> fa1/1(in1)
  Bit_Slice_79/1 -> fa26/2(in2)
  fa29/2(C) -> Concat_1/2
  Bit_Slice_75/1 -> fa25/1(in1)
  fa8/1(S) -> Concat/24
  Bit_Slice_90/1 -> fa30/1(in1)
  fa18/2(C) -> Concat_1/13
  fa7/2(C) -> Concat_1/24
  fa30/1(S) -> Concat/2
  Bit_Slice_31/1 -> fa10/2(in2)
  fa25/2(C) -> Concat_1/6
  Bit_Slice_89/1 -> fa29/3(Cin)
  Bit_Slice_91/1 -> fa30/2(in2)
  fa9/2(C) -> Concat_1/22
  fa11/1(S) -> Concat/21
  fa18/1(S) -> Concat/14
  Bit_Slice_72/1 -> fa24/1(in1)
  fa22/2(C) -> Concat_1/9
  fa24/2(C) -> Concat_1/7
  Bit_Slice_82/1 -> fa27/2(in2)
  fa28/2(C) -> Concat_1/3
  fa25/1(S) -> Concat/7
  Bit_Slice_58/1 -> fa19/2(in2)
  Bit_Slice_6/1 -> fa2/1(in1)
  Bit_Slice_87/1 -> fa29/1(in1)
  Bit_Slice/1 -> fa/1(in1)
  fa10/2(C) -> Concat_1/21
  fa28/1(S) -> Concat/4
  Bit_Slice_88/1 -> fa29/2(in2)
  fa24/1(S) -> Concat/8
  Bit_Slice_76/1 -> fa25/2(in2)
  fa16/2(C) -> Concat_1/15
  Bit_Slice_20/1 -> fa6/3(Cin)
  Bit_Slice_28/1 -> fa9/2(in2)
  Bit_Slice_80/1 -> fa26/3(Cin)
  Bit_Slice_84/1 -> fa28/1(in1)
  Bit_Slice_43/1 -> fa14/2(in2)
  Bit_Slice_55/1 -> fa18/2(in2)
  fa23/1(S) -> Concat/9
  Concat_1/1 -> C/1
  Bit_Slice_71/1 -> fa23/3(Cin)
  fa22/1(S) -> Concat/10
  Bit_Slice_65/1 -> fa21/3(Cin)
  Bit_Slice_49/1 -> fa16/2(in2)
  Bit_Slice_4/1 -> fa1/2(in2)
  Bit_Slice_70/1 -> fa23/2(in2)
  Bit_Slice_68/1 -> fa22/3(Cin)
  in3/1 -> Bit_Slice_92/1, Bit_Slice_89/1, Bit_Slice_86/1, Bit_Slice_83/1, Bit_Slice_80/1, Bit_Slice_77/1, Bit_Slice_74/1, Bit_Slice_71/1, Bit_Slice_68/1, Bit_Slice_65/1, Bit_Slice_62/1, Bit_Slice_59/1, Bit_Slice_56/1, Bit_Slice_53/1, Bit_Slice_50/1, Bit_Slice_47/1, Bit_Slice_44/1, Bit_Slice_41/1, Bit_Slice_38/1, Bit_Slice_35/1, Bit_Slice_32/1, Bit_Slice_29/1, Bit_Slice_26/1, Bit_Slice_23/1, Bit_Slice_20/1, Bit_Slice_17/1, Bit_Slice_14/1, Bit_Slice_11/1, Bit_Slice_8/1, Bit_Slice_5/1, Bit_Slice_2/1
  fa13/2(C) -> Concat_1/18
  Bit_Slice_67/1 -> fa22/2(in2)
  fa13/1(S) -> Concat/19
  fa21/2(C) -> Concat_1/10
  Bit_Slice_53/1 -> fa17/3(Cin)
  Bit_Slice_26/1 -> fa8/3(Cin)
  fa21/1(S) -> Concat/11
  Bit_Slice_63/1 -> fa21/1(in1)
  Bit_Slice_27/1 -> fa9/1(in1)
  fa20/2(C) -> Concat_1/11
  fa20/1(S) -> Concat/12
  fa17/2(C) -> Concat_1/14
  Bit_Slice_60/1 -> fa20/1(in1)
  Bit_Slice_62/1 -> fa20/3(Cin)
  Bit_Slice_38/1 -> fa12/3(Cin)
  Bit_Slice_61/1 -> fa20/2(in2)
  fa19/1(S) -> Concat/13
  Bit_Slice_11/1 -> fa3/3(Cin)
  Bit_Slice_69/1 -> fa23/1(in1)
  Bit_Slice_66/1 -> fa22/1(in1)
  Bit_Slice_59/1 -> fa19/3(Cin)
  Bit_Slice_56/1 -> fa18/3(Cin)
  Bit_Slice_54/1 -> fa18/1(in1)
  fa17/1(S) -> Concat/15
  Bit_Slice_51/1 -> fa17/1(in1)
  Bit_Slice_52/1 -> fa17/2(in2)
  fa16/1(S) -> Concat/16
  Bit_Slice_50/1 -> fa16/3(Cin)
  Bit_Slice_48/1 -> fa16/1(in1)
  fa15/2(C) -> Concat_1/16
  in2/1 -> Bit_Slice_91/1, Bit_Slice_88/1, Bit_Slice_85/1, Bit_Slice_82/1, Bit_Slice_79/1, Bit_Slice_76/1, Bit_Slice_73/1, Bit_Slice_70/1, Bit_Slice_67/1, Bit_Slice_64/1, Bit_Slice_61/1, Bit_Slice_58/1, Bit_Slice_55/1, Bit_Slice_52/1, Bit_Slice_49/1, Bit_Slice_46/1, Bit_Slice_43/1, Bit_Slice_40/1, Bit_Slice_37/1, Bit_Slice_34/1, Bit_Slice_31/1, Bit_Slice_28/1, Bit_Slice_25/1, Bit_Slice_22/1, Bit_Slice_19/1, Bit_Slice_16/1, Bit_Slice_13/1, Bit_Slice_10/1, Bit_Slice_7/1, Bit_Slice_4/1, Bit_Slice_1/1
  Bit_Slice_36/1 -> fa12/1(in1)
  fa15/1(S) -> Concat/17
  fa19/2(C) -> Concat_1/12
  Bit_Slice_47/1 -> fa15/3(Cin)
